simulink model "Four_DoF_03_prismatic"  (R2024a)
settings: Solver=ode1be  StartTime=0.0  StopTime=inf  FixedStep=0.001  RelTol=1e-3
undefined symbols (not defined in the file or in its folder): X, Y, Z
libraries: sm_lib x62, nesl_utility x21, robotcorelib x4
(part 1 of 3)
settings Model: Creator=Chaiyapat Gotji  LastModifiedBy=pimna
settings RTWCC: GPUComputeCapability=3.5

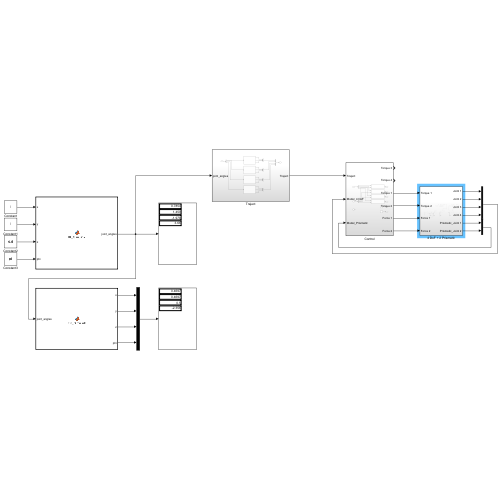
[thumbnail: Simulink's stored preview of the top-level diagram]
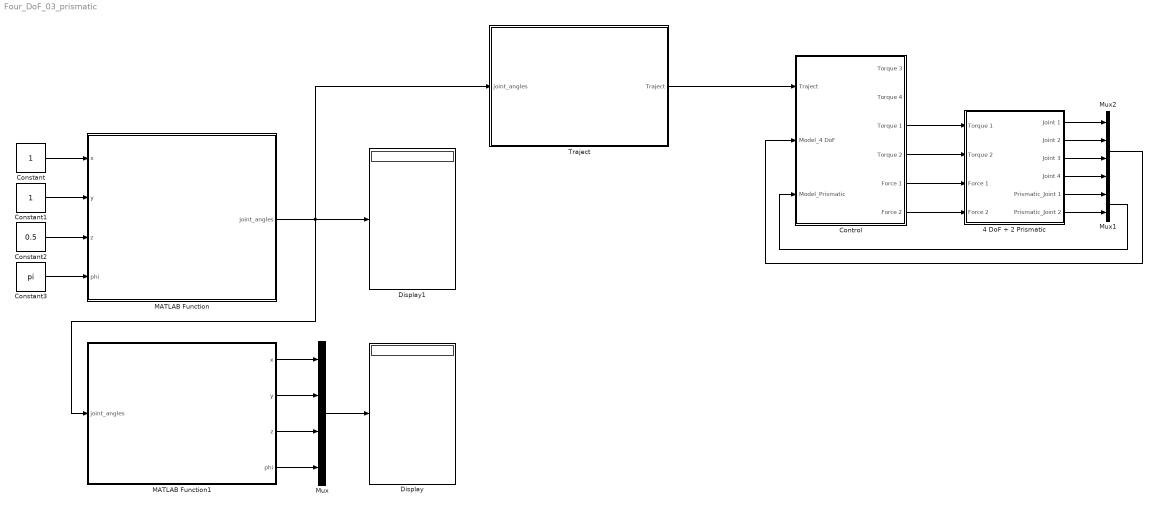
== system Four_DoF_03_prismatic ==
  4 DoF + 2 Prismatic : Subsystem
  Constant : Constant  VectorParams1D=off  SampleTime=-1
  Constant1 : Constant  VectorParams1D=off  SampleTime=-1
  Constant2 : Constant  Value=0.5  VectorParams1D=off  SampleTime=-1
  Constant3 : Constant  Value=pi  VectorParams1D=off  SampleTime=-1
  Control : Subsystem
  Display : Display
  Display1 : Display
  MATLAB Function : MATLAB Function  TreatAsAtomicUnit=on
  MATLAB Function1 : MATLAB Function  TreatAsAtomicUnit=on
  Mux : Mux
  Mux1 : Mux  Inputs=2
  Mux2 : Mux
  Traject : Subsystem
  wires:
  Mux2/1 -> Control/2(Model_4 DoF)
  Traject/1(Traject) -> Control/1(Traject)
  Control/3(Torque 1) -> 4 DoF + 2 Prismatic/1(Torque 1)
  Control/4(Torque 2) -> 4 DoF + 2 Prismatic/2(Torque 2)
  4 DoF + 2 Prismatic/1(Joint 1) -> Mux2/1
  4 DoF + 2 Prismatic/2(Joint 2) -> Mux2/2
  4 DoF + 2 Prismatic/3(Joint 3) -> Mux2/3
  4 DoF + 2 Prismatic/4(Joint 4) -> Mux2/4
  4 DoF + 2 Prismatic/5(Prismatic_Joint 1) -> Mux1/1
  4 DoF + 2 Prismatic/6(Prismatic_Joint 2) -> Mux1/2
  Mux1/1 -> Control/3(Model_Prismatic)
  Control/5(Force 1) -> 4 DoF + 2 Prismatic/3(Force 1)
  Control/6(Force 2) -> 4 DoF + 2 Prismatic/4(Force 2)
  Constant/1 -> MATLAB Function/1(x)
  Constant1/1 -> MATLAB Function/2(y)
  Constant2/1 -> MATLAB Function/3(z)
  Constant3/1 -> MATLAB Function/4(phi)
  MATLAB Function1/1(x) -> Mux/1
  MATLAB Function1/2(y) -> Mux/2
  MATLAB Function1/3(z) -> Mux/3
  MATLAB Function1/4(phi) -> Mux/4
  Mux/1 -> Display/1
  MATLAB Function/1(joint_angles) -> MATLAB Function1/1(joint_angles), Traject/1(joint_angles), Display1/1
